simulink model "nonlinearxsystemController2"  (R2020b)
settings: Solver=VariableStepAuto  StartTime=0.0  StopTime=10.0  RelTol=1e-3
settings Model: Creator=Javad  LastModifiedBy=Javad

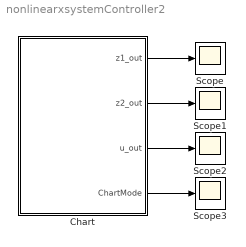
== system nonlinearxsystemController2 ==
  Chart : Stateflow chart  TreatAsAtomicUnit=on
  Scope{,1..3} (4 alike) : Scope
  wires:
  Chart/3(u_out) -> Scope2/1
  Chart/2(z2_out) -> Scope1/1
  Chart/1(z1_out) -> Scope/1
  Chart/4(ChartMode) -> Scope3/1

== stateflow chart nonlinearxsystemController2/Chart ==
  settings: updateMethod=CONTINUOUS
  state Q2
    du:
    z1_dot=-30*z1-20*z2+24+20*(1.261*z1-8.527*z2-0.2);
    z2_dot=0.05*z1-50*(-2*0.001*z2+1.4*0.001);
    z1_out=z1;
    z2_out=z2;
    u_out=1.261*z1-8.527*z2-0.2;
  state Q1
    du:
    z1_dot=-30*z1-20*z2+24+20*(1.339*z1-7.067*z2+0.2);
    z2_dot=0.05*z1-50*(5*0.001*z2);
    z1_out=z1;
    z2_out=z2;
    u_out=1.339*z1-7.067*z2+0.2;
  state Q3
    du:
    z1_dot=-30*z1-20*z2+24+20*(1.310*z1-10.547*z2);
    z2_dot=0.05*z1-50*(4*0.001*z2-2.2*0.001);
    z1_out=z1;
    z2_out=z2;
    u_out=1.310*z1-10.547*z2;
  (default) -> Q1 : {z1=0.5;
      | z2=0.1;}
  Q2 -> Q1 [order 2] : [z2<0.2]
  Q1 -> Q2 : [z2>=0.2]
  Q2 -> Q3 [order 1] : [z2>=0.6]
  Q3 -> Q2 : [z2<0.6]
  data: z1_out output; z2_out output; u_out output; z2 local; z1 local; x1_eq constant double =0.3714; x2_eq constant double =0.6429; ChartMode output Enum: ChartModeType
  data z2 settings: updateMethod=SF_CONTINUOUS_TIME_DATA
  data z1 settings: updateMethod=SF_CONTINUOUS_TIME_DATA
